simulink model "mgr_sim"  (R2016a)
settings: Solver=FixedStepAuto  StartTime=0.0  StopTime=10.0  FixedStep=0.01  RelTol=1e-3
values from neighbouring files (symbols this model uses):
  alpha = alpha_v(i)    [mgr.m]
  beta = alpha/10    [mgr.m]
  check_start = radio_stop    (= 50)    [mgr.m]
  check_stop = check_start+step    (= 51)    [mgr.m]
  chemo_on = 1    [mgr.m]
  cis_days = [0 28]    [mgr.m]
  cis_det = step/cis_hl    (= 0.1)    [mgr.m]
  cis_dose = 0.1*surface    (= 0.17)    [mgr.m]
  death_cond = death_cond*5.8e8    (= 667200975794)    [mgr.m]
  gamma = 0.0093    [mgr.m]
  K = K*5.8e8    (= 8.19955682587e+12)    [mgr.m]
  model = 0    [mgr.m]
  N_in = N_in*5.8e8    (= 65596454607)    [mgr.m]
  radio_amp = radio_dose/radio_duration    (= 1.28571428571)    [mgr.m]
  radio_on = 1    [mgr.m]
  radio_start = 1    [mgr.m]
  radio_stop = radio_start+radio_duration    (= 50)    [mgr.m]
  ro = ro_v(i)    [mgr.m]
  ro_e = 3*ro    [mgr.m]
  ro_m = met_scale*ro    [mgr.m]
  ro_m_e = met_scale*ro_e    [mgr.m]
  t_m = normrnd(20, 10)    [mgr.m]
  vin_days = [0 7 14 21 28]    [mgr.m]
  vin_dose = 0.05*surface*0.4    (= 0.034)    [mgr.m]
libraries: simulink x1
settings Model: Creator=TOSHIBA  LastModifiedBy=TOSHIBA

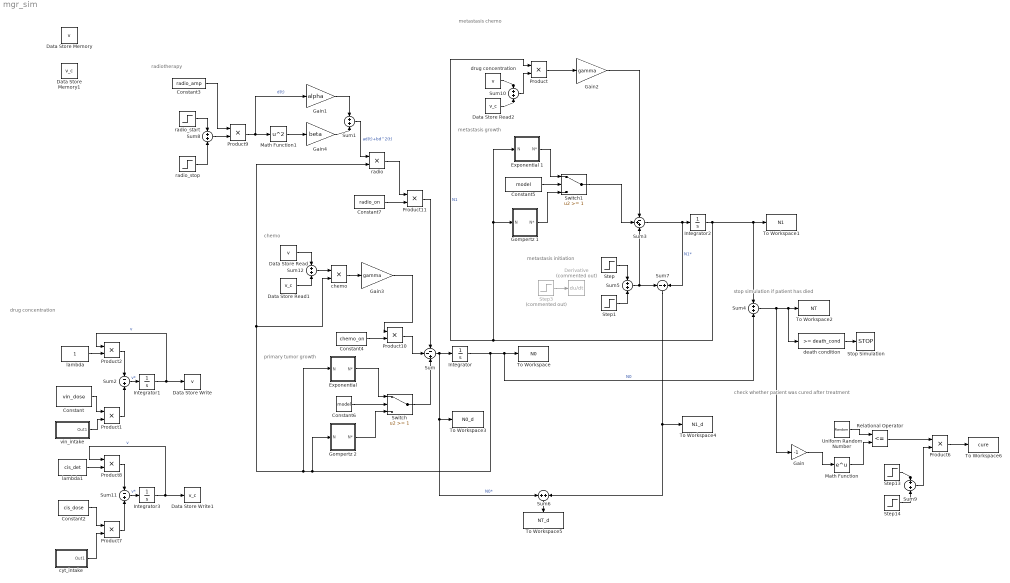
== system mgr_sim ==
  note: stop simulation if patient has died
  note: check whether patient was cured after treatment
  note: metastasis chemo
  note: metastasis initiation
  note: metastasis growth
  note: primary tumor growth
  note: chemo
  note: drug concentration
  note: radiotherapy
  Constant : Constant  Value=vin_dose
  Constant2 : Constant  Value=cis_dose
  Constant3 : Constant  Value=radio_amp
  Constant4 : Constant  Value=chemo_on
  Constant5 : Constant  Value=model
  Constant6 : Constant  Value=model
  Constant7 : Constant  Value=radio_on
  Data Store Memory : DataStoreMemory  DataStoreName=v  ReadBeforeWriteMsg=warning  WriteAfterWriteMsg=warning  WriteAfterReadMsg=warning  ShowAdditionalParam=off
  Data Store Memory1 : DataStoreMemory  DataStoreName=v_c  ReadBeforeWriteMsg=warning  WriteAfterWriteMsg=warning  WriteAfterReadMsg=warning  ShowAdditionalParam=off
  Data Store Read : DataStoreRead  DataStoreName=v
  Data Store Read1 : DataStoreRead  DataStoreName=v_c
  Data Store Read2 : DataStoreRead  DataStoreName=v_c
  Data Store Write : DataStoreWrite  DataStoreName=v
  Data Store Write1 : DataStoreWrite  DataStoreName=v_c
  Derivative : Derivative  Commented=on
  "Exponential " : Subsystem
  Exponential 1 : Subsystem
  Gain : Gain  Gain=-1
  Gain1 : Gain  Gain=alpha
  Gain2 : Gain  Gain=gamma
  Gain3 : Gain  Gain=gamma
  Gain4 : Gain  Gain=beta
  Gompertz 1 : Subsystem
  Gompertz 2 : Subsystem
  Integrator : Integrator  InitialCondition=N_in
  Integrator1 : Integrator
  Integrator2 : Integrator
  Integrator3 : Integrator
  Math Function : Math  SaturateOnIntegerOverflow=on
  Math Function1 : Math  Operator=square  SaturateOnIntegerOverflow=on
  Product{,1..2,6..11} (9 alike) : Product
  Relational Operator : RelationalOperator  Operator=<=  OutDataTypeStr=boolean
  Step : Step  Time=t_m  After=1000  SampleTime=0
  Step1 : Step  Time=t_m+step  After=-1000  SampleTime=0
  Step13 : Step  Time=check_start  SampleTime=0
  Step14 : Step  Time=check_stop  After=-1  SampleTime=0
  Step3 : Step  Commented=on  SampleTime=0
  Stop Simulation : Stop
  Sum : Sum  Inputs=--+
  Sum{1,4..6,8..10,12} (8 alike) : Sum
  Sum11 : Sum  Inputs=-+
  Sum2 : Sum  Inputs=-+
  Sum3 : Sum  Inputs=-++
  Sum7 : Sum  Inputs=-+
  Switch : Switch  Threshold=1
  Switch1 : Switch  Threshold=1
  To Workspace : ToWorkspace  VariableName=N0  SaveFormat=Timeseries  SampleTime=-1
  To Workspace1 : ToWorkspace  VariableName=N1  SaveFormat=Timeseries  SampleTime=-1
  To Workspace2 : ToWorkspace  VariableName=NT  SaveFormat=Timeseries  SampleTime=-1
  To Workspace3 : ToWorkspace  VariableName=N0_d  SaveFormat=Timeseries  SampleTime=-1
  To Workspace4 : ToWorkspace  VariableName=N1_d  SaveFormat=Timeseries  SampleTime=-1
  To Workspace5 : ToWorkspace  VariableName=NT_d  SaveFormat=Timeseries  SampleTime=-1
  To Workspace6 : ToWorkspace  VariableName=cure  SaveFormat=Timeseries  SampleTime=-1
  Uniform Random Number : UniformRandomNumber  Minimum=0  SampleTime=1
  chemo : Product
  cyt_intake : Subsystem
  death condition : simulink/Logic and Bit Operations/Compare To Constant  relop=>=  const=death_cond  OutDataTypeStr=boolean
  drug concentration : DataStoreRead  DataStoreName=v
  lambda : Constant
  lambda1 : Constant  Value=cis_det
  radio : Product
  radio_start : Step  Time=radio_start  SampleTime=0
  radio_stop : Step  Time=radio_stop  After=-1  SampleTime=0
  vin_intake : Subsystem
  wires:
  Sum/1 -> Sum6/1, To Workspace3/1, Integrator/1  "N0*"
  Sum1/1 -> radio/1  "ad(t)+bd^2(t)"
  Integrator1/1 -> Data Store Write/1, Product2/1  "v"
  Sum2/1 -> Integrator1/1  "v*"
  Product2/1 -> Sum2/1
  Math Function1/1 -> Gain4/1
  Product9/1 -> Gain1/1, Math Function1/1  "d(t)"
  Sum3/1 -> Sum7/2, Integrator2/1  "N1*"
  Sum4/1 -> Gain/1, death condition/1, To Workspace2/1
  lambda/1 -> Product2/2
  "Exponential "/1(N*) -> Switch/1
  Switch/1 -> Sum/3
  Constant6/1 -> Switch/2
  Gompertz 2/1(N*) -> Switch/3
  Integrator2/1 -> Gompertz 1/1(N), Exponential 1/1(N), Product/1, To Workspace1/1, Sum4/1  "N1"
  Exponential 1/1(N*) -> Switch1/1
  Gompertz 1/1(N*) -> Switch1/3
  Constant5/1 -> Switch1/2
  Step/1 -> Sum5/1
  Sum5/1 -> Sum3/3, Sum7/1
  Step1/1 -> Sum5/2
  Step3/1 -> Derivative/1
  death condition/1 -> Stop Simulation/1
  Sum6/1 -> To Workspace5/1
  Sum7/1 -> To Workspace4/1, Sum6/2
  Constant/1 -> Product1/1
  Integrator/1 -> Gompertz 2/1(N), "Exponential "/1(N), chemo/2, radio/2, Sum4/2, To Workspace/1  "N0"
  Switch1/1 -> Sum3/2
  Product/1 -> Gain2/1
  Gain/1 -> Math Function/1
  Uniform Random Number/1 -> Relational Operator/1
  Math Function/1 -> Relational Operator/2
  Relational Operator/1 -> Product6/1
  Product6/1 -> To Workspace6/1
  Sum9/1 -> Product6/2
  Step13/1 -> Sum9/1
  Step14/1 -> Sum9/2
  Product1/1 -> Sum2/2
  Constant2/1 -> Product7/1
  Integrator3/1 -> Data Store Write1/1, Product8/1  "v"
  Sum11/1 -> Integrator3/1  "v*"
  Product8/1 -> Sum11/1
  lambda1/1 -> Product8/2
  Product7/1 -> Sum11/2
  Data Store Read/1 -> Sum12/1
  Sum12/1 -> chemo/1
  Data Store Read1/1 -> Sum12/2
  radio_stop/1 -> Sum8/2
  radio_start/1 -> Sum8/1
  Constant3/1 -> Product9/1
  Sum8/1 -> Product9/2
  vin_intake/1(Out1) -> Product1/2
  cyt_intake/1(Out1) -> Product7/2
  Product10/1 -> Sum/2
  Product11/1 -> Sum/1
  radio/1 -> Product11/1
  Constant7/1 -> Product11/2
  drug concentration/1 -> Sum10/1
  Data Store Read2/1 -> Sum10/2
  Constant4/1 -> Product10/2
  chemo/1 -> Gain3/1
  Gain1/1 -> Sum1/1
  Sum10/1 -> Product/2
  Gain2/1 -> Sum3/1
  Gain3/1 -> Product10/1
  Gain4/1 -> Sum1/2

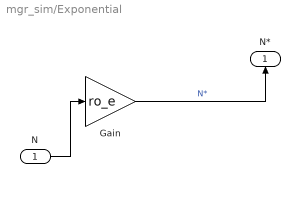
== system mgr_sim/Exponential  ==
  N : Inport
  Gain : Gain  Gain=ro_e
  N* : Outport
  wires:
  Gain/1 -> N*/1  "N*"
  N/1 -> Gain/1

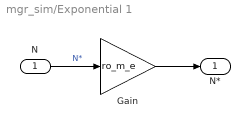
== system mgr_sim/Exponential 1 ==
  N : Inport
  Gain : Gain  Gain=ro_m_e
  N* : Outport
  wires:
  N/1 -> Gain/1  "N*"
  Gain/1 -> N*/1

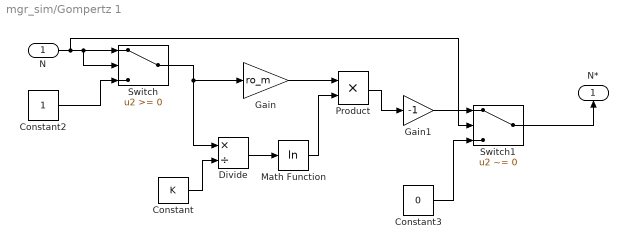
== system mgr_sim/Gompertz 1 ==
  N : Inport
  Constant : Constant  Value=K
  Constant2 : Constant
  Constant3 : Constant  Value=0
  Divide : Product  Inputs=*/
  Gain : Gain  Gain=ro_m
  Gain1 : Gain  Gain=-1
  Math Function : Math  Operator=log  SaturateOnIntegerOverflow=on
  Product : Product
  Switch : Switch
  Switch1 : Switch  Criteria=u2 ~= 0
  N* : Outport
  wires:
  Switch/1 -> Divide/1, Gain/1
  Constant/1 -> Divide/2
  Divide/1 -> Math Function/1
  Product/1 -> Gain1/1
  N/1 -> Switch1/2, Switch/2, Switch/1
  Constant2/1 -> Switch/3
  Switch1/1 -> N*/1
  Constant3/1 -> Switch1/3
  Gain/1 -> Product/1
  Gain1/1 -> Switch1/1
  Math Function/1 -> Product/2

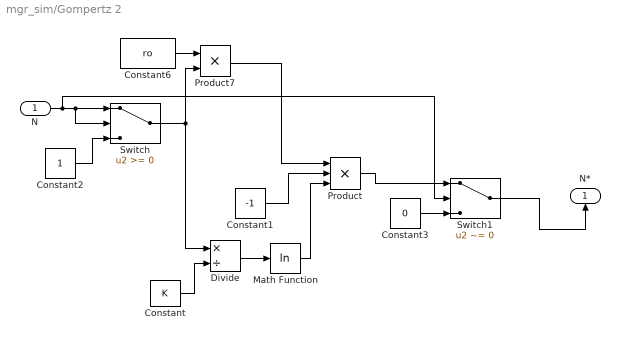
== system mgr_sim/Gompertz 2 ==
  N : Inport
  Constant : Constant  Value=K
  Constant1 : Constant  Value=-1
  Constant2 : Constant
  Constant3 : Constant  Value=0
  Constant6 : Constant  Value=ro
  Divide : Product  Inputs=*/
  Math Function : Math  Operator=log  SaturateOnIntegerOverflow=on
  Product : Product  Inputs=3
  Product7 : Product
  Switch : Switch
  Switch1 : Switch  Criteria=u2 ~= 0
  N* : Outport
  wires:
  Constant6/1 -> Product7/1
  Switch/1 -> Product7/2, Divide/1
  Constant/1 -> Divide/2
  Divide/1 -> Math Function/1
  Math Function/1 -> Product/3
  Product7/1 -> Product/1
  Product/1 -> Switch1/1
  N/1 -> Switch1/2, Switch/2, Switch/1
  Constant2/1 -> Switch/3
  Switch1/1 -> N*/1
  Constant3/1 -> Switch1/3
  Constant1/1 -> Product/2

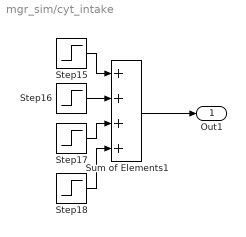
== system mgr_sim/cyt_intake ==
  Step15 : Step  Time=cis_days(1)+step  SampleTime=0
  Step16 : Step  Time=cis_days(1)+step  After=-1  SampleTime=0
  Step17 : Step  Time=cis_days(2)  SampleTime=0
  Step18 : Step  Time=cis_days(2)+step  After=-1  SampleTime=0
  Sum of Elements1 : Sum  Inputs=++++
  Out1 : Outport
  wires:
  Step17/1 -> Sum of Elements1/3
  Sum of Elements1/1 -> Out1/1
  Step15/1 -> Sum of Elements1/1
  Step16/1 -> Sum of Elements1/2
  Step18/1 -> Sum of Elements1/4

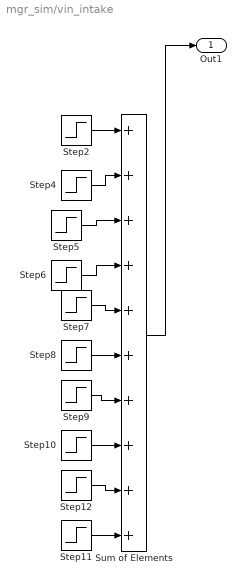
== system mgr_sim/vin_intake ==
  Step10 : Step  Time=28+step  After=-1  SampleTime=0
  Step11 : Step  Time=35+step  After=-1  SampleTime=0
  Step12 : Step  Time=35  SampleTime=0
  Step2 : Step  Time=vin_days(1)  SampleTime=0
  Step4 : Step  Time=7+step  After=-1  SampleTime=0
  Step5 : Step  Time=14  SampleTime=0
  Step6 : Step  Time=14+step  After=-1  SampleTime=0
  Step7 : Step  Time=21  SampleTime=0
  Step8 : Step  Time=21+step  After=-1  SampleTime=0
  Step9 : Step  Time=28  SampleTime=0
  Sum of Elements : Sum  Inputs=++++++++++
  Out1 : Outport
  wires:
  Step2/1 -> Sum of Elements/1
  Sum of Elements/1 -> Out1/1
  Step7/1 -> Sum of Elements/5
  Step8/1 -> Sum of Elements/6
  Step12/1 -> Sum of Elements/9
  Step4/1 -> Sum of Elements/2
  Step5/1 -> Sum of Elements/3
  Step6/1 -> Sum of Elements/4
  Step10/1 -> Sum of Elements/8
  Step9/1 -> Sum of Elements/7
  Step11/1 -> Sum of Elements/10
